simulink model "untitled"  (R2024b)
settings: Solver=VariableStepAuto  StartTime=0.0  StopTime=10.0  RelTol=1e-3
settings Model: Creator=Asus TUF  LastModifiedBy=Asus TUF

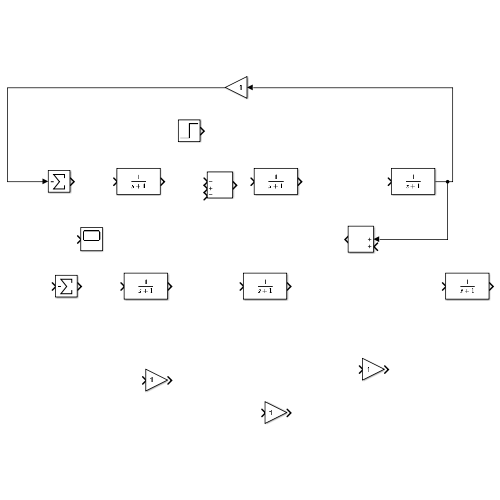
[thumbnail: Simulink's stored preview of the top-level diagram]
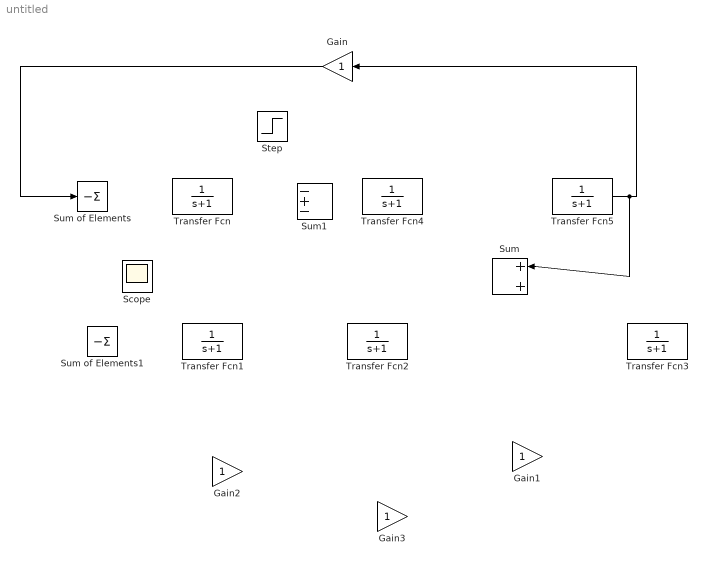
== system untitled ==
  Gain{,1..3} (4 alike) : Gain
  Scope : Scope
  Step : Step  SampleTime=0
  Sum : Sum  Inputs=|++
  Sum of Elements : Sum  Inputs=-
  Sum of Elements1 : Sum  Inputs=-
  Sum1 : Sum  Inputs=|-+-
  Transfer Fcn{,1..5} (6 alike) : TransferFcn  Denominator=[1 1]
  wires:
  Gain/1 -> Sum of Elements/1
  Transfer Fcn5/1 -> Sum/1, Gain/1
